simulink model "sf"  (Simulink 6.4)
settings: Solver=ode45  StartTime=0.0  StopTime=tm  MaxStep=tr  RelTol=1e-3
values from neighbouring files (symbols this model uses):
  B = 52.2786    [mechanical_example.m]
  k = 113832    [mechanical_example.m]
  M = 12.5 * 0.45359237    (= 5.669904625)    [mechanical_example.m]
settings Model: Creator=christopher.rappa  LastModifiedBy=michael.sangillo
settings OptimizationCC: InlineInvariantSignals=on
settings DebuggingCC: StrictBusMsg=None

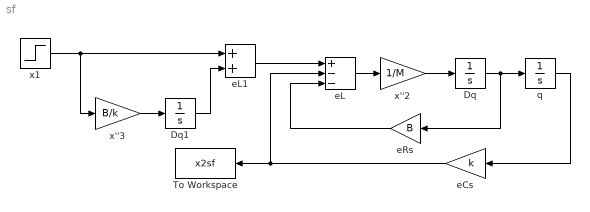
== system sf ==
  Dq : Integrator
  Dq1 : Integrator
  To Workspace : ToWorkspace  VariableName=x2sf  SampleTime=-1  SaveFormat=Structure With Time
  eCs : Gain  Orientation=left  Gain=k
  eL : Sum  Inputs=+--  OutScaling=2^-10
  eL1 : Sum  OutScaling=2^-10
  eRs : Gain  Orientation=left  Gain=B
  q : Integrator
  x''2 : Gain  Gain=1/M
  x''3 : Gain  Gain=B/k
  x1 : Step  Time=0  SampleTime=0
  wires:
  q/1 -> eCs/1
  eCs/1 -> eL/2, To Workspace/1
  Dq/1 -> q/1, eRs/1
  eRs/1 -> eL/3
  eL/1 -> x''2/1
  x''2/1 -> Dq/1
  x1/1 -> x''3/1, eL1/1
  eL1/1 -> eL/1
  x''3/1 -> Dq1/1
  Dq1/1 -> eL1/2
